simulink model "SimuHybrid_Ex1"  (R2024a)
settings: Solver=VariableStepAuto  StartTime=ti  StopTime=tf  FixedStep=dt  MaxStep=1e-3  RelTol=1e-4  AbsTol=1e-6
values from neighbouring files (symbols this model uses):
  doffset = 0    [LaunchSimulation.m]
  dperiod = 0.5    [LaunchSimulation.m]
settings Model: Creator=perruquetti  LastModifiedBy=perruquetti
settings SolverCC: AlgebraicLoopSolver=LineSearch
settings DebuggingCC: AlgebraicLoopMsg=none  UnconnectedInputMsg=warning  UnconnectedOutputMsg=warning  UnconnectedLineMsg=warning
settings ModelReferenceCC: EnableRefExpFcnMdlSchedulingChecks=on
settings RTWCC: GPUComputeCapability=3.5  DLArmComputeVersion=19.05

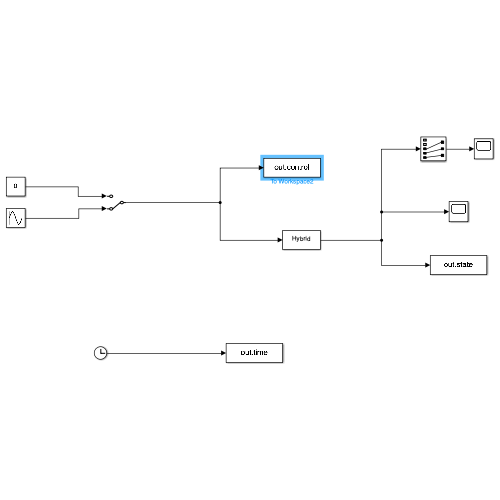
[thumbnail: Simulink's stored preview of the top-level diagram]
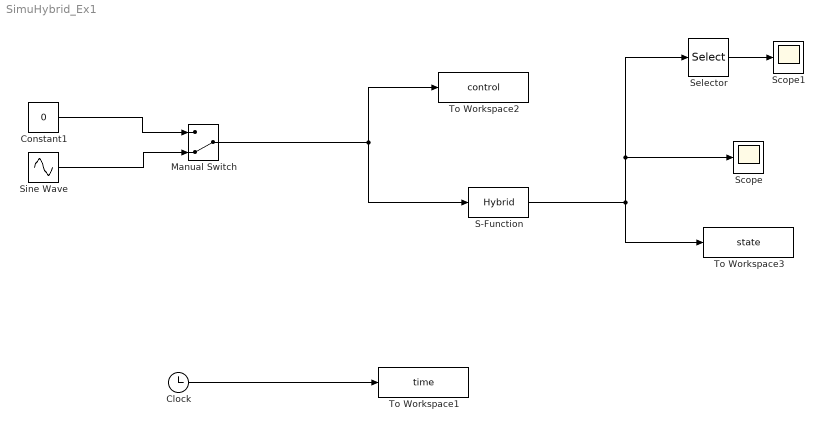
== system SimuHybrid_Ex1 ==
  Clock : Clock
  Constant1 : Constant  Value=0
  Manual Switch : ManualSwitch  CurrentSetting=0
  S-Function : S-Function  FunctionName=Hybrid  Parameters=dperiod,doffset  SFunctionDeploymentMode=off  EnableBusSupport=off
  Scope : Scope
  Scope1 : Scope
  Selector : Selector  InputPortWidth=5  IndexOptions=Index vector (dialog)  Indices=[3 4 5]  OutputSizes=1
  Sine Wave : Sin  SampleTime=0
  To Workspace1 : ToWorkspace  VariableName=time  SampleTime=-1
  To Workspace2 : ToWorkspace  VariableName=control  SaveFormat=Structure With Time  SampleTime=-1
  To Workspace3 : ToWorkspace  VariableName=state  SaveFormat=Structure With Time  SampleTime=-1
  wires:
  Clock/1 -> To Workspace1/1
  S-Function/1 -> Scope/1, Selector/1, To Workspace3/1
  Constant1/1 -> Manual Switch/1
  Sine Wave/1 -> Manual Switch/2
  Manual Switch/1 -> S-Function/1, To Workspace2/1
  Selector/1 -> Scope1/1
